simulink model "NonlinearBlockCustomObserver"  (R2019b)
settings: Solver=VariableStepAuto  StartTime=0.0  StopTime=10.0  RelTol=1e-3
libraries: eeLuenbergerObserver x2
settings Model: Creator=marko  LastModifiedBy=marko

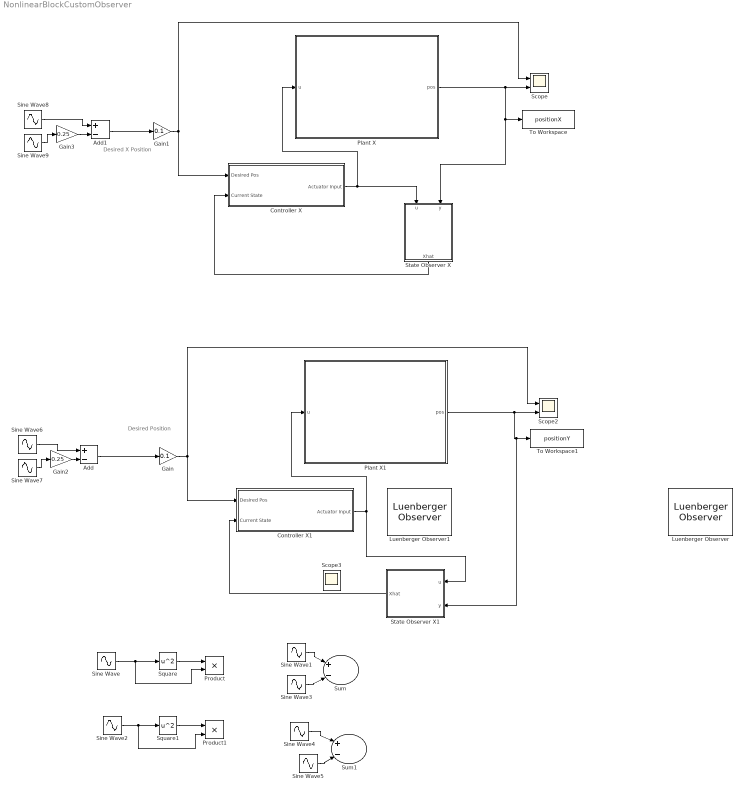
== system NonlinearBlockCustomObserver ==
  note: Desired X Position
  note: Desired Position
  Add : Sum  Inputs=+-
  Add1 : Sum  Inputs=+-
  Controller X : Subsystem
  Controller X1 : Subsystem
  Gain : Gain  Gain=0.1
  Gain1 : Gain  Gain=0.1
  Gain2 : Gain  Gain=0.25
  Gain3 : Gain  Gain=0.25
  Luenberger Observer : eeLuenbergerObserver/Luenberger Observer  StateSpaceType=Continuous-time  Ad=1  Bd=1  Cd=1  Dd=1  A=[0 1 0 0; 0 -1 -9.8 0; 0 0 0 1; -0.98/(0.33) 0 0 -0.1/(0.33)]  B=[0; 0; 0; 3]  C=[1 0 0 0]  D=0  ObserverDesign=Desired eigenvalues  Ld=1  DesiredEigenvalues=[-40, -50, -60, -70]  x0=[0; 0; 0; 0]  Tsd=0.01  Ts=0.01
      settings: SourceProductName=Simscape Electrical  SourceProductBaseCode=PS
  Luenberger Observer1 : eeLuenbergerObserver/Luenberger Observer  StateSpaceType=Continuous-time  Ad=1  Bd=1  Cd=1  Dd=1  A=[0 1 0 0; 0 -1 -9.8 0; 0 0 0 1; -0.98/(0.33) 0 0 -0.1/(0.33)]  B=[0; 0; 0; 3]  C=[1 0 0 0]  D=0  ObserverDesign=Desired eigenvalues  Ld=1  DesiredEigenvalues=[-40, -50, -60, -70]  x0=[0; 0; 0; 0]  Tsd=0.01  Ts=0.01
      settings: SourceProductName=Simscape Electrical  SourceProductBaseCode=PS
  Plant X : Subsystem
  Plant X1 : Subsystem
  Product : Product
  Product1 : Product
  Scope : Scope  NumInputPorts=2
  Scope2 : Scope  NumInputPorts=2
  Scope3 : Scope  NumInputPorts=2
  Sine Wave : Sin  SampleTime=0
  Sine Wave1 : Sin  Amplitude=2  SampleTime=0
  Sine Wave2 : Sin  Phase=pi/2  SampleTime=0
  Sine Wave3 : Sin  Frequency=2  SampleTime=0
  Sine Wave4 : Sin  Amplitude=2  Phase=pi/2  SampleTime=0
  Sine Wave5 : Sin  Frequency=2  Phase=pi/2  SampleTime=0
  Sine Wave6 : Sin  Amplitude=1.25  SampleTime=0
  Sine Wave7 : Sin  Frequency=5  SampleTime=0
  Sine Wave8 : Sin  Amplitude=1.25  Phase=pi/2  SampleTime=0
  Sine Wave9 : Sin  Frequency=5  Phase=pi/2  SampleTime=0
  Square : Math  Operator=square  SignedPower=off  SaturateOnIntegerOverflow=on
  Square1 : Math  Operator=square  SignedPower=off  SaturateOnIntegerOverflow=on
  State Observer X : Subsystem
  State Observer X1 : Subsystem
  Sum : Sum  Inputs=|+-|
  Sum1 : Sum  Inputs=|+-|
  To Workspace : ToWorkspace  VariableName=positionX  SampleTime=-1
  To Workspace1 : ToWorkspace  VariableName=positionY  SampleTime=-1
  wires:
  Plant X/1(pos) -> Scope/2, To Workspace/1, State Observer X/2(y)
  Add1/1 -> Gain1/1
  Sine Wave4/1 -> Sum1/1
  Sine Wave3/1 -> Sum/2
  Sine Wave1/1 -> Sum/1
  Sine Wave5/1 -> Sum1/2
  Controller X/1(Actuator Input) -> Plant X/1(u), State Observer X/1(u)
  Add/1 -> Gain/1
  Controller X1/1(Actuator Input) -> Plant X1/1(u), State Observer X1/1(u)
  Plant X1/1(pos) -> Scope2/2, State Observer X1/2(y), To Workspace1/1
  Gain3/1 -> Add1/2
  Sine Wave8/1 -> Add1/1
  Sine Wave9/1 -> Gain3/1
  Sine Wave7/1 -> Gain2/1
  Sine Wave6/1 -> Add/1
  Gain2/1 -> Add/2
  Gain/1 -> Scope2/1, Controller X1/1(Desired Pos)
  Gain1/1 -> Scope/1, Controller X/1(Desired Pos)
  State Observer X/1(Xhat) -> Controller X/2(Current State)
  State Observer X1/1(Xhat) -> Controller X1/2(Current State)
  Square/1 -> Product/1
  Sine Wave/1 -> Product/2, Square/1
  Sine Wave2/1 -> Product1/2, Square1/1
  Square1/1 -> Product1/1

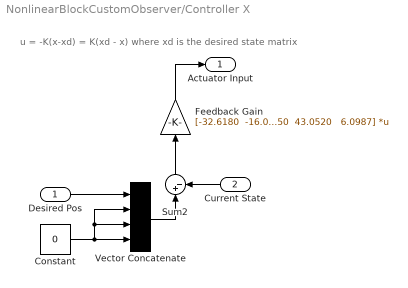
== system NonlinearBlockCustomObserver/Controller X ==
  note: u = -K(x-xd) = K(xd - x) where xd is the desired state matrix
  Desired Pos : Inport
  Current State : Inport  Port=2
  Constant : Constant  Value=0
  Feedback Gain : Gain  Gain="[-32.6180  -16.0550  43.0520   6.0987]"  Multiplication=Matrix(K*u)
  Sum2 : Sum  Inputs=|+-
  Vector Concatenate : Concatenate  NumInputs=4
  Actuator Input : Outport
  wires:
  Desired Pos/1 -> Vector Concatenate/1
  Feedback Gain/1 -> Actuator Input/1
  Constant/1 -> Vector Concatenate/2, Vector Concatenate/3, Vector Concatenate/4
  Current State/1 -> Sum2/2
  Sum2/1 -> Feedback Gain/1
  Vector Concatenate/1 -> Sum2/1

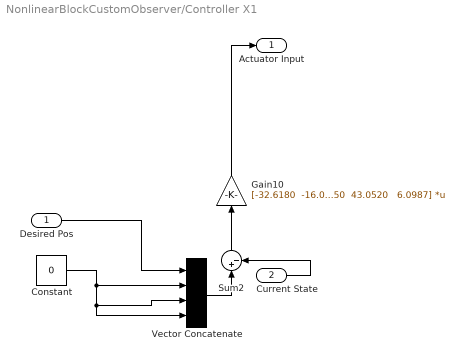
== system NonlinearBlockCustomObserver/Controller X1 ==
  Desired Pos : Inport
  Current State : Inport  Port=2
  Constant : Constant  Value=0
  Gain10 : Gain  Gain="[-32.6180  -16.0550  43.0520   6.0987]"  Multiplication=Matrix(K*u)
  Sum2 : Sum  Inputs=|+-
  Vector Concatenate : Concatenate  NumInputs=4
  Actuator Input : Outport
  wires:
  Desired Pos/1 -> Vector Concatenate/1
  Gain10/1 -> Actuator Input/1
  Constant/1 -> Vector Concatenate/2, Vector Concatenate/4, Vector Concatenate/3
  Current State/1 -> Sum2/2
  Sum2/1 -> Gain10/1
  Vector Concatenate/1 -> Sum2/1

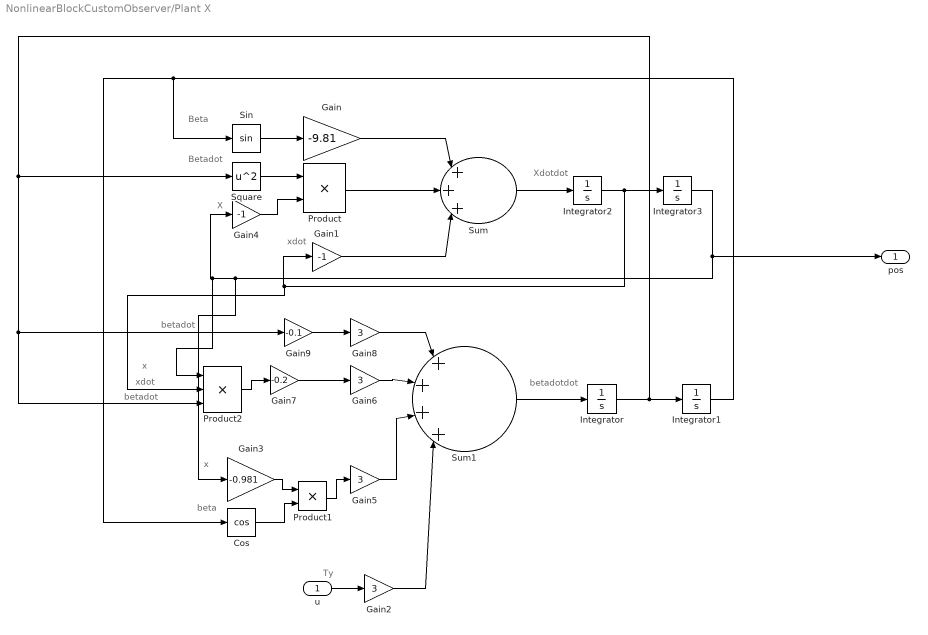
== system NonlinearBlockCustomObserver/Plant X ==
  note: betadotdot
  note: betadot
  note: betadot
  note: xdot
  note: x
  note: beta
  note: x
  note: Ty
  note: xdot
  note: X
  note: Betadot
  note: Beta
  note: Xdotdot
  u : Inport
  Cos : Trigonometry  Operator=cos
  Gain : Gain  Gain=-9.81
  Gain1 : Gain  Gain=-1
  Gain{2,5..6,8} (4 alike) : Gain  Gain=3
  Gain3 : Gain  Gain=-0.981
  Gain4 : Gain  Gain=-1
  Gain7 : Gain  Gain=-0.2
  Gain9 : Gain  Gain=-0.1
  Integrator{,1..3} (4 alike) : Integrator
  Product : Product
  Product1 : Product
  Product2 : Product  Inputs=3
  Sin : Trigonometry
  Square : Math  Operator=square  SignedPower=off  SaturateOnIntegerOverflow=on
  Sum : Sum  Inputs=|+++|
  Sum1 : Sum  Inputs=|++++|
  pos : Outport
  wires:
  Gain2/1 -> Sum1/4
  Gain8/1 -> Sum1/1
  Sum1/1 -> Integrator/1
  Integrator3/1 -> pos/1, Gain3/1, Product2/1, Gain4/1
  Product1/1 -> Gain5/1
  Gain1/1 -> Sum/3
  Product/1 -> Sum/2
  Gain4/1 -> Product/2
  Sum/1 -> Integrator2/1
  Square/1 -> Product/1
  Gain3/1 -> Product1/1
  Gain6/1 -> Sum1/2
  Gain9/1 -> Gain8/1
  Gain/1 -> Sum/1
  Cos/1 -> Product1/2
  Integrator/1 -> Gain9/1, Product2/3, Square/1, Integrator1/1
  Integrator1/1 -> Cos/1, Sin/1
  Gain5/1 -> Sum1/3
  Gain7/1 -> Gain6/1
  Sin/1 -> Gain/1
  Integrator2/1 -> Product2/2, Gain1/1, Integrator3/1
  Product2/1 -> Gain7/1
  u/1 -> Gain2/1

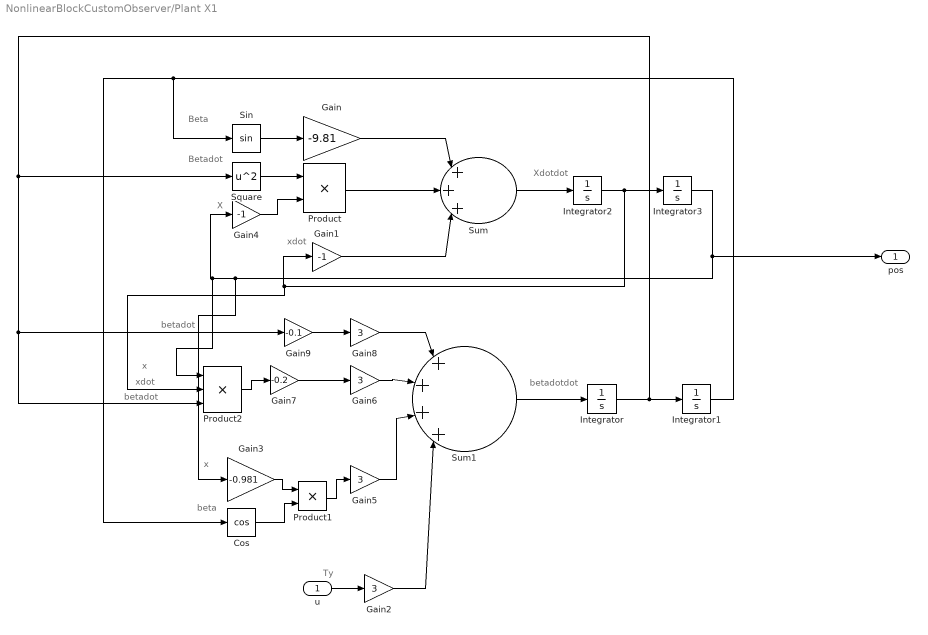
== system NonlinearBlockCustomObserver/Plant X1 ==
  note: betadotdot
  note: betadot
  note: betadot
  note: xdot
  note: x
  note: beta
  note: x
  note: Ty
  note: xdot
  note: X
  note: Betadot
  note: Beta
  note: Xdotdot
  u : Inport
  Cos : Trigonometry  Operator=cos
  Gain : Gain  Gain=-9.81
  Gain1 : Gain  Gain=-1
  Gain{2,5..6,8} (4 alike) : Gain  Gain=3
  Gain3 : Gain  Gain=-0.981
  Gain4 : Gain  Gain=-1
  Gain7 : Gain  Gain=-0.2
  Gain9 : Gain  Gain=-0.1
  Integrator{,1..3} (4 alike) : Integrator
  Product : Product
  Product1 : Product
  Product2 : Product  Inputs=3
  Sin : Trigonometry
  Square : Math  Operator=square  SignedPower=off  SaturateOnIntegerOverflow=on
  Sum : Sum  Inputs=|+++|
  Sum1 : Sum  Inputs=|++++|
  pos : Outport
  wires:
  Gain2/1 -> Sum1/4
  Gain8/1 -> Sum1/1
  Sum1/1 -> Integrator/1
  Integrator3/1 -> pos/1, Gain3/1, Product2/1, Gain4/1
  Product1/1 -> Gain5/1
  Gain1/1 -> Sum/3
  Product/1 -> Sum/2
  Gain4/1 -> Product/2
  Sum/1 -> Integrator2/1
  Square/1 -> Product/1
  Gain3/1 -> Product1/1
  Gain6/1 -> Sum1/2
  Gain9/1 -> Gain8/1
  Gain/1 -> Sum/1
  Cos/1 -> Product1/2
  Integrator/1 -> Gain9/1, Product2/3, Square/1, Integrator1/1
  Integrator1/1 -> Cos/1, Sin/1
  Gain5/1 -> Sum1/3
  Gain7/1 -> Gain6/1
  Sin/1 -> Gain/1
  Integrator2/1 -> Product2/2, Gain1/1, Integrator3/1
  Product2/1 -> Gain7/1
  u/1 -> Gain2/1

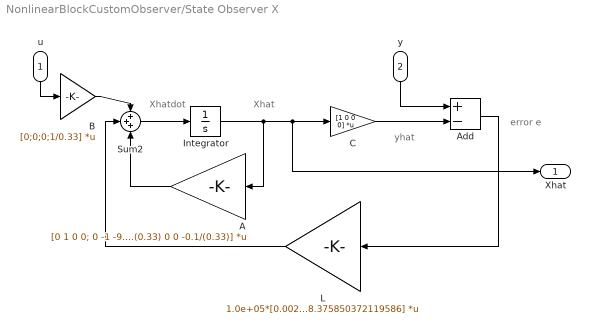
== system NonlinearBlockCustomObserver/State Observer X ==
  note: Xhat
  note: error e
  note: yhat
  note: Xhatdot
  u : Inport
  y : Inport  Port=2
  A : Gain  Gain=[0 1 0 0; 0 -1 -9.8 0; 0 0 0 1; -0.98/(0.33) 0 0 -0.1/(0.33)]  Multiplication=Matrix(K*u)
  Add : Sum  Inputs=+-
  B : Gain  Gain=[0;0;0;1/0.33]  Multiplication=Matrix(K*u)
  C : Gain  Gain=[1 0 0 0]  Multiplication=Matrix(K*u)
  Integrator : Integrator  InitialCondition=[0;0;0;0]
  L : Gain  Gain=1.0e+05*[0.002186969696867;0.176147281894242; -0.645506052740811;-8.375850372119586]  Multiplication=Matrix(K*u)
  Sum2 : Sum  Inputs=+++
  Xhat : Outport
  wires:
  B/1 -> Sum2/1
  L/1 -> Sum2/2
  Integrator/1 -> A/1, C/1, Xhat/1
  Sum2/1 -> Integrator/1
  A/1 -> Sum2/3
  u/1 -> B/1
  C/1 -> Add/2
  y/1 -> Add/1
  Add/1 -> L/1

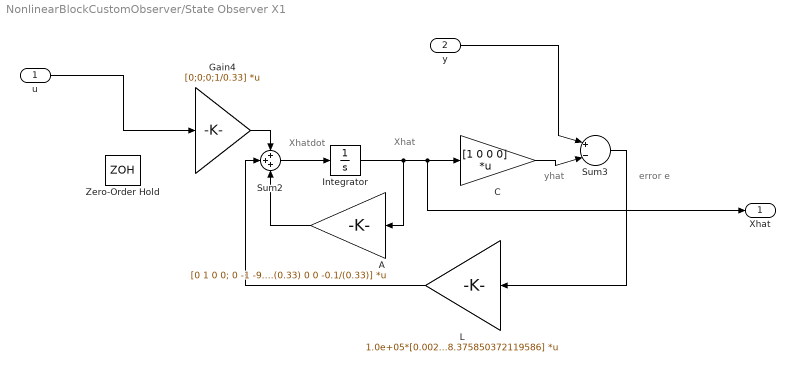
== system NonlinearBlockCustomObserver/State Observer X1 ==
  note: Xhat
  note: error e
  note: yhat
  note: Xhatdot
  u : Inport
  y : Inport  Port=2
  A : Gain  Gain=[0 1 0 0; 0 -1 -9.8 0; 0 0 0 1; -0.98/(0.33) 0 0 -0.1/(0.33)]  Multiplication=Matrix(K*u)
  C : Gain  Gain=[1 0 0 0]  Multiplication=Matrix(K*u)
  Gain4 : Gain  Gain=[0;0;0;1/0.33]  Multiplication=Matrix(K*u)
  Integrator : Integrator  InitialCondition=[0;0;0;0]
  L : Gain  Gain=1.0e+05*[0.002186969696867;0.176147281894242; -0.645506052740811;-8.375850372119586]  Multiplication=Matrix(K*u)
  Sum2 : Sum  Inputs=+++
  Sum3 : Sum  Inputs=|+-|
  Zero-Order Hold : ZeroOrderHold  SampleTime=0.01
  Xhat : Outport
  wires:
  Gain4/1 -> Sum2/1
  L/1 -> Sum2/2
  Integrator/1 -> A/1, Xhat/1, C/1
  C/1 -> Sum3/2
  Sum3/1 -> L/1
  Sum2/1 -> Integrator/1
  A/1 -> Sum2/3
  u/1 -> Gain4/1
  y/1 -> Sum3/1
